simulink model "AssegnamentoAutovalori"  (R2025b)
settings: Solver=VariableStepAuto  StartTime=0.0  StopTime=10.0  RelTol=1e-3
undefined symbols (not defined in the file): A, B, C, C_EIG, D, K_EIG, N, x0_EIG, x_ref
settings Model: Creator=salvo  LastModifiedBy=salvo

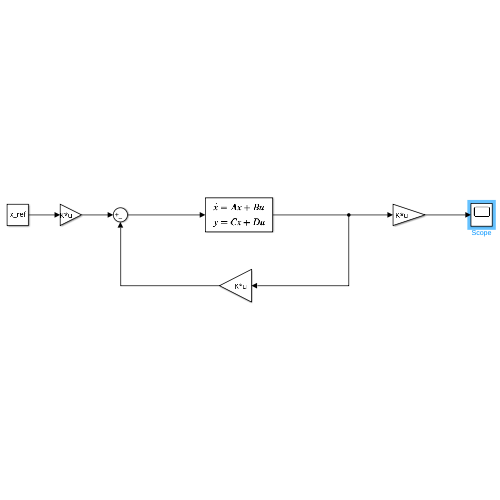
[thumbnail: Simulink's stored preview of the top-level diagram]
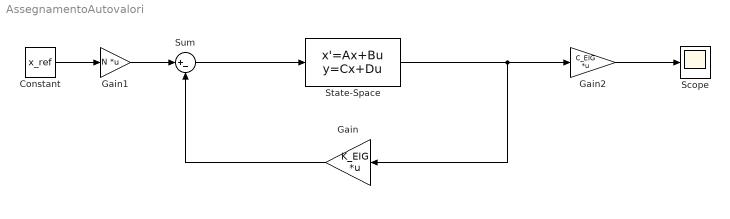
== system AssegnamentoAutovalori ==
  Constant : Constant  Value=x_ref
  Gain : Gain  Gain=K_EIG  Multiplication=Matrix(K*u)
  Gain1 : Gain  Gain=N  Multiplication=Matrix(K*u)
  Gain2 : Gain  Gain=C_EIG  Multiplication=Matrix(K*u)
  Scope : Scope
      settings: ActiveDisplayYMinimum=0.24383151458436594  ActiveDisplayYMaximum=0.6678321828164917
  State-Space : StateSpace  A=A  B=B  C=C  D=D  InitialCondition=x0_EIG
  Sum : Sum  Inputs=|+-
  wires:
  State-Space/1 -> Gain2/1, Gain/1
  Sum/1 -> State-Space/1
  Gain/1 -> Sum/2
  Gain1/1 -> Sum/1
  Constant/1 -> Gain1/1
  Gain2/1 -> Scope/1
